simulink model "motor"  (R2020b)
settings: Solver=ode45  StartTime=0.0  StopTime=23  RelTol=1e-3  EnableMultiTasking=on
PreLoadFcn:
  | MotorParam
InitFcn:
  | MotorParam
values from neighbouring files (symbols this model uses):
  B = (Km*INL)/w    (= 4.14319136746e-07)    [MotorParam.m]
  J = Rotor_inertia    (= 2.23668e-07)    [MotorParam.m]
  Kb = (Speed_constant)/(.10472)    (= 0.0177826336223)    [MotorParam.m]
  Km = Torque_constant*1E-3    (= 0.0178)    [MotorParam.m]
  L = Terminal_inductance*1E-3    (= 0.000411)    [MotorParam.m]
  R = Terminal_resistance    (= 5.82)    [MotorParam.m]
libraries: simulink x1
settings Model: Creator=Leo  LastModifiedBy=Jeff
settings DataIOCC: LimitDataPoints=on  SaveFormat=Array  SignalLoggingSaveFormat=ModelDataLogs  ReturnWorkspaceOutputs=off
settings OptimizationCC: ExpressionDepthLimit=2147483647  InitFltsAndDblsToZero=on  LifeSpan=inf
settings DebuggingCC: UnderspecifiedInitializationDetection=Classic  MergeDetectMultiDrivingBlocksExec=none  SolverPrmCheckMsg=warning  FcnCallInpInsideContextMsg=warning  StateNameClashWarn=warning  SFUnexpectedBacktrackingDiag=warning  SFNoUnconditionalDefaultTransitionDiag=warning  SFExecutionAtInitializationDiag=none  ArithmeticOperatorsInVariantConditions=warning
settings HardwareCC: ProdBitPerPointer=32  ProdBitPerSizeT=32  ProdBitPerPtrDiffT=32  ProdLargestAtomicFloat=None  ProdIntDivRoundTo=Undefined  ProdEndianess=Unspecified  ProdWordSize=32  ProdHWDeviceType=32-bit Generic
settings ModelReferenceCC: PropagateSignalLabelsOutOfModel=off
settings SFSimCC: SimUseLocalCustomCode=off  CustomCodeUndefinedFunction=UseInterfaceOnly
settings RTWCC: RTWUseLocalCustomCode=off
settings CodeAppCC: StateflowObjectComments=on
settings GRTTargetCC: TargetLangStandard=C89/C90 (ANSI)  CombineOutputUpdateFcns=off  GRTInterface=on
settings ConfigComp: CovMetricSettings=dw  CovSaveCumulativeToWorkspaceVar=on  CovSaveSingleToWorkspaceVar=on  CovExternalEMLEnable=off  CovSFcnEnable=off

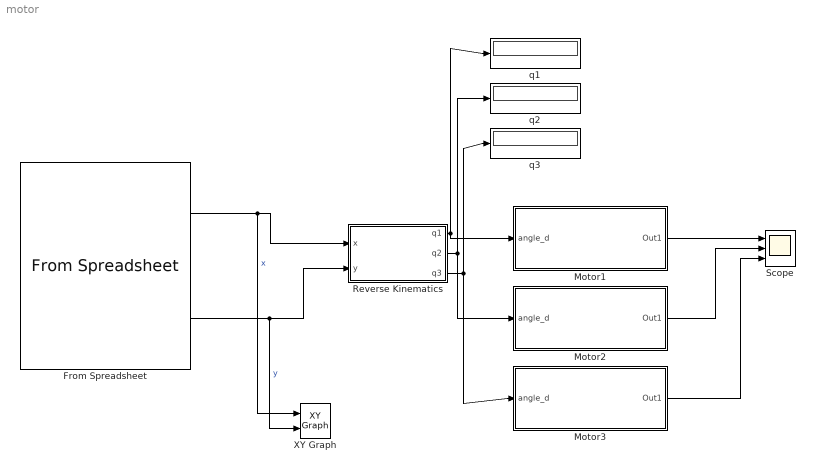
== system motor ==
  From Spreadsheet : FromSpreadsheet  FileName=Motor_pos.xlsx
  Motor1 : Subsystem
  Motor2 : Subsystem
  Motor3 : Subsystem
  Reverse Kinematics : MATLAB Function  TreatAsAtomicUnit=on
  Scope : Scope  NumInputPorts=3
  XY Graph : simulink/Sinks/XY Graph  xmin=-15  xmax=15  ymin=-5  ymax=50  st=0.001
  q1 : Display
  q2 : Display
  q3 : Display
  wires:
  From Spreadsheet/1 -> XY Graph/1, Reverse Kinematics/1(x)  "x"
  Motor1/1(Out1) -> Scope/1
  From Spreadsheet/2 -> XY Graph/2, Reverse Kinematics/2(y)  "y"
  Reverse Kinematics/1(q1) -> q1/1, Motor1/1(angle_d)
  Reverse Kinematics/2(q2) -> Motor2/1(angle_d), q2/1
  Reverse Kinematics/3(q3) -> Motor3/1(angle_d), q3/1
  Motor2/1(Out1) -> Scope/2
  Motor3/1(Out1) -> Scope/3

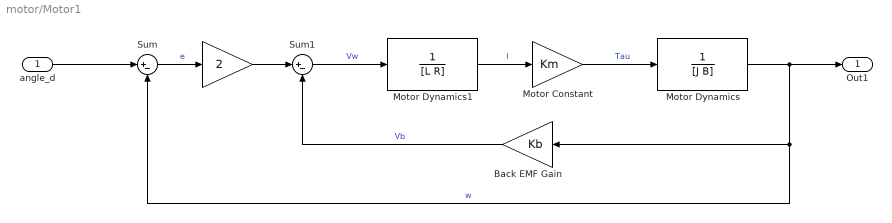
== system motor/Motor1 ==
  angle_d : Inport
  " " : Gain  Gain=2
  Back EMF Gain : Gain  Gain=Kb
  Motor Constant : Gain  Gain=Km
  Motor Dynamics : TransferFcn  Denominator=[J B]
  Motor Dynamics1 : TransferFcn  Denominator=[L R]
  Sum : Sum  Inputs=|+-
  Sum1 : Sum  Inputs=|+-
  Out1 : Outport
  wires:
  angle_d/1 -> Sum/1
  Sum/1 -> " "/1  "e"
  Motor Dynamics/1 -> Out1/1, Sum/2, Back EMF Gain/1  "w"
  Motor Constant/1 -> Motor Dynamics/1  "Tau"
  " "/1 -> Sum1/1
  Back EMF Gain/1 -> Sum1/2  "Vb"
  Motor Dynamics1/1 -> Motor Constant/1  "I"
  Sum1/1 -> Motor Dynamics1/1  "Vw"

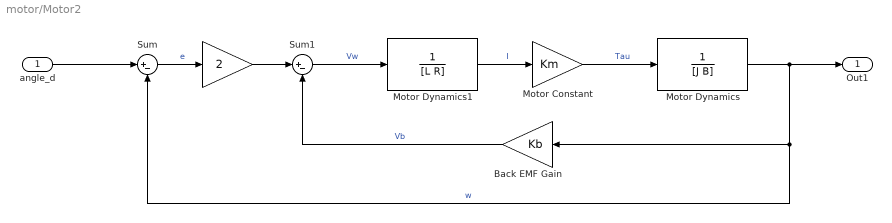
== system motor/Motor2 ==
  angle_d : Inport
  " " : Gain  Gain=2
  Back EMF Gain : Gain  Gain=Kb
  Motor Constant : Gain  Gain=Km
  Motor Dynamics : TransferFcn  Denominator=[J B]
  Motor Dynamics1 : TransferFcn  Denominator=[L R]
  Sum : Sum  Inputs=|+-
  Sum1 : Sum  Inputs=|+-
  Out1 : Outport
  wires:
  angle_d/1 -> Sum/1
  Sum/1 -> " "/1  "e"
  Motor Dynamics/1 -> Out1/1, Sum/2, Back EMF Gain/1  "w"
  Motor Constant/1 -> Motor Dynamics/1  "Tau"
  " "/1 -> Sum1/1
  Back EMF Gain/1 -> Sum1/2  "Vb"
  Motor Dynamics1/1 -> Motor Constant/1  "I"
  Sum1/1 -> Motor Dynamics1/1  "Vw"

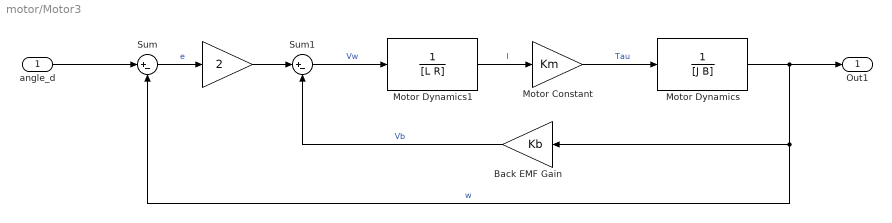
== system motor/Motor3 ==
  angle_d : Inport
  " " : Gain  Gain=2
  Back EMF Gain : Gain  Gain=Kb
  Motor Constant : Gain  Gain=Km
  Motor Dynamics : TransferFcn  Denominator=[J B]
  Motor Dynamics1 : TransferFcn  Denominator=[L R]
  Sum : Sum  Inputs=|+-
  Sum1 : Sum  Inputs=|+-
  Out1 : Outport
  wires:
  angle_d/1 -> Sum/1
  Sum/1 -> " "/1  "e"
  Motor Dynamics/1 -> Out1/1, Sum/2, Back EMF Gain/1  "w"
  Motor Constant/1 -> Motor Dynamics/1  "Tau"
  " "/1 -> Sum1/1
  Back EMF Gain/1 -> Sum1/2  "Vb"
  Motor Dynamics1/1 -> Motor Constant/1  "I"
  Sum1/1 -> Motor Dynamics1/1  "Vw"

== matlab function motor/Reverse Kinematics ==
  data: x input; q1 output; y input; q2 output; q3 output
    function [q1, q2, q3]= fcn(x,y)
    a1 = 20;
    a2 = 30;
    
    q2 = acosd((x^2+y^2-a1^2-a2^2)/(2*a1*a2));
    q1 = atand(y/x)-atand(a2*sind(q2)/(a1+a2*cosd(q2)));
    if q1<0 
        q1 = 180+q1;
    end
    q3 = 180-q1-q2;
    if q3<0
        q3 = 90;
    end
